simulink model "IncisionDicison"  (R2023a)
settings: Solver=FixedStepAuto  StartTime=0.0  StopTime=inf  RelTol=1e-3  EnableMultiTasking=on
libraries: vexarmcortexlib x24, vexcommonlib x7
settings Model: ExtModeTrigDuration=25  Creator=bobsi  LastModifiedBy=bobsi
settings OptimizationCC: EnhancedBackFolding=on  PassReuseOutputArgsAs=Individual arguments  ZeroExternalMemoryAtStartup=off  ZeroInternalMemoryAtStartup=off  MaxStackSize=64  OptimizeBlockOrder=speed  DifferentSizesBufferReuse=on  OptimizationCustomize=off  EfficientTunableParamExpr=on
settings DebuggingCC: ParameterTunabilityLossMsg=error
settings HardwareCC: ProdBitPerPointer=32  ProdBitPerSizeT=32  ProdBitPerPtrDiffT=32  ProdLargestAtomicInteger=Long  ProdLargestAtomicFloat=Double  ProdWordSize=32  ProdHWDeviceType=ARM Compatible->ARM Cortex
settings SFSimCC: MATLABDynamicMemAlloc=off
settings RTWCC: Description=Embedded Coder  SystemTargetFile=ert.tlc  HardwareBoard=ARM Cortex-based VEX Microcontroller  TLCOptions="-aInlineSetEventsForThisBaseRateFcn=TLC_FALSE -aSuppressMultiTaskScheduler=TLC_FALSE  -aRateBasedStepFcn=0"  TemplateMakefile=ert_default_tmf  Toolchain=GNU Tools for VEX ARM Cortex
settings CodeAppCC: ForceParamTrailComments=on  IgnoreCustomStorageClasses=off  OperatorAnnotations=on  SimulinkDataObjDesc=on  SFDataObjDesc=on  InsertBlockDesc=on
settings ERTTargetCC: ExtModeTransport=1  ExtModeMexFile=ext_serial_win32_comm

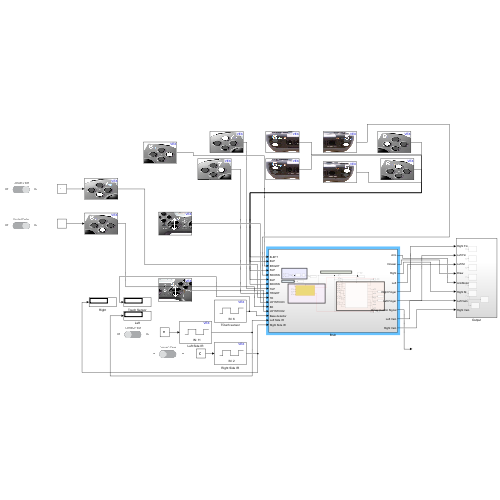
[thumbnail: Simulink's stored preview of the top-level diagram]
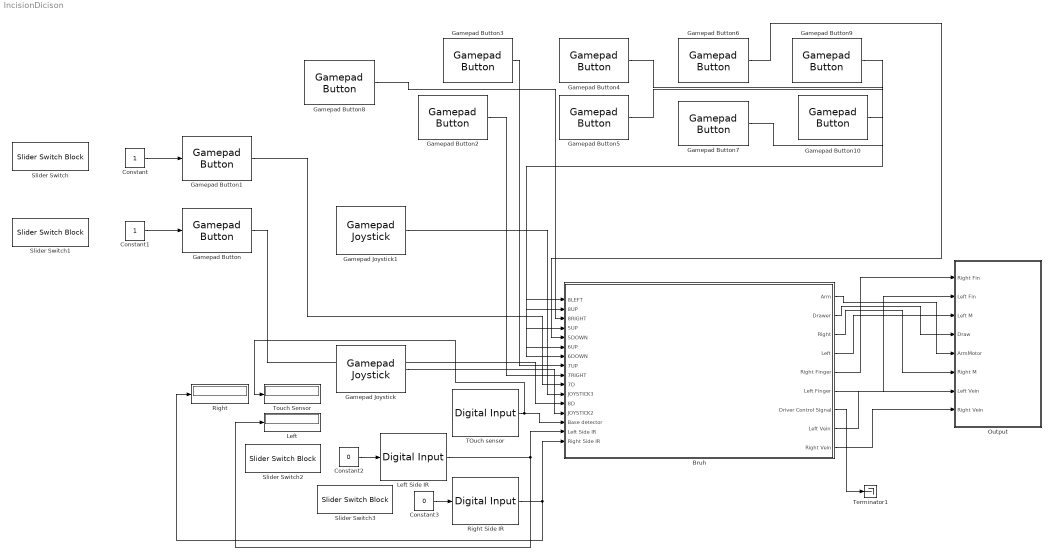
== system IncisionDicison ==
  Bruh : Subsystem
  Constant : Constant
  Constant1 : Constant
  Constant2 : Constant  Value=0
  Constant3 : Constant  Value=0
  Gamepad Button : vexarmcortexlib/Gamepad/Gamepad Button  joystick=1  chan=8  button56=Up  button78=Down  SimulationIn=on  SampleTime=0.02
  Gamepad Button1 : vexarmcortexlib/Gamepad/Gamepad Button  joystick=1  chan=7  button56=Up  button78=Down  SimulationIn=on  SampleTime=0.02
  Gamepad Button10 : vexarmcortexlib/Gamepad/Gamepad Button  joystick=1  chan=8  button56=Up  button78=Up  SimulationIn=off  SampleTime=0.02
  Gamepad Button2 : vexarmcortexlib/Gamepad/Gamepad Button  joystick=1  chan=7  button56=Up  button78=Right  SimulationIn=off  SampleTime=0.02
  Gamepad Button3 : vexarmcortexlib/Gamepad/Gamepad Button  joystick=1  chan=7  button56=Up  button78=Up  SimulationIn=off  SampleTime=0.02
  Gamepad Button4 : vexarmcortexlib/Gamepad/Gamepad Button  joystick=1  chan=6  button56=Down  button78=Down  SimulationIn=off  SampleTime=0.02
  Gamepad Button5 : vexarmcortexlib/Gamepad/Gamepad Button  joystick=1  chan=6  button56=Up  button78=Down  SimulationIn=off  SampleTime=0.02
  Gamepad Button6 : vexarmcortexlib/Gamepad/Gamepad Button  joystick=1  chan=5  button56=Down  button78=Down  SimulationIn=off  SampleTime=0.02
  Gamepad Button7 : vexarmcortexlib/Gamepad/Gamepad Button  joystick=1  chan=5  button56=Up  button78=Down  SimulationIn=off  SampleTime=0.02
  Gamepad Button8 : vexarmcortexlib/Gamepad/Gamepad Button  joystick=1  chan=8  button56=Up  button78=Right  SimulationIn=off  SampleTime=0.02
  Gamepad Button9 : vexarmcortexlib/Gamepad/Gamepad Button  joystick=1  chan=8  button56=Up  button78=Left  SimulationIn=off  SampleTime=0.02
  Gamepad Joystick : vexarmcortexlib/Gamepad/Gamepad Joystick  joystick=1  chan=2  SimulationIn=off  SampleTime=0.02
  Gamepad Joystick1 : vexarmcortexlib/Gamepad/Gamepad Joystick  joystick=1  chan=3  SimulationIn=off  SampleTime=0.02
  Left : Display
  Left Side IR : vexarmcortexlib/Sensors/Digital Input  inChan=11  SimulationIn=on  SampleTime=0.02
  Output : Subsystem
  Right : Display
  Right Side IR : vexarmcortexlib/Sensors/Digital Input  inChan=2  SimulationIn=on  SampleTime=0.02
  Slider Switch{,1..3} (4 alike) : SliderSwitchBlock
      settings: Values={{'Off', 'On'}, [0 1]}
  TOuch sensor : vexarmcortexlib/Sensors/Digital Input  inChan=6  SimulationIn=off  SampleTime=0.02
  Terminator1 : Terminator
  Touch Sensor : Display
  wires:
  Bruh/3(Right) -> Output/6(Right M)
  Bruh/6(Left Finger) -> Output/2(Left Fin)
  Bruh/5(Right Finger) -> Output/1(Right Fin)
  Bruh/4(Left) -> Output/3(Left M)
  Bruh/2(Drawer) -> Output/4(Draw)
  Bruh/1(Arm) -> Output/5(ArmMotor)
  Bruh/7(Driver Control Signal) -> Terminator1/1
  Right Side IR/1 -> Right/1, Bruh/16(Right Side IR)
  Left Side IR/1 -> Left/1, Bruh/15(Left Side IR)
  TOuch sensor/1 -> Touch Sensor/1, Bruh/14(Base detector)
  Gamepad Joystick/1 -> Bruh/13(JOYSTICK2)
  Gamepad Button/1 -> Bruh/12(8D)
  Gamepad Joystick1/1 -> Bruh/11(JOYSTICK3)
  Gamepad Button1/1 -> Bruh/10(7D)
  Gamepad Button2/1 -> Bruh/9(7RIGHT)
  Gamepad Button3/1 -> Bruh/8(7UP)
  Gamepad Button4/1 -> Bruh/7(6DOWN)
  Gamepad Button5/1 -> Bruh/6(6UP)
  Gamepad Button6/1 -> Bruh/5(5DOWN)
  Gamepad Button7/1 -> Bruh/4(5UP)
  Gamepad Button8/1 -> Bruh/3(8RIGHT)
  Gamepad Button10/1 -> Bruh/2(8UP)
  Gamepad Button9/1 -> Bruh/1(8LEFT)
  Bruh/8(Left Vein) -> Output/7(Left Vein)
  Bruh/9(Right Vein) -> Output/8(Right Vein)
  Constant/1 -> Gamepad Button1/1
  Constant1/1 -> Gamepad Button/1
  Constant2/1 -> Left Side IR/1
  Constant3/1 -> Right Side IR/1

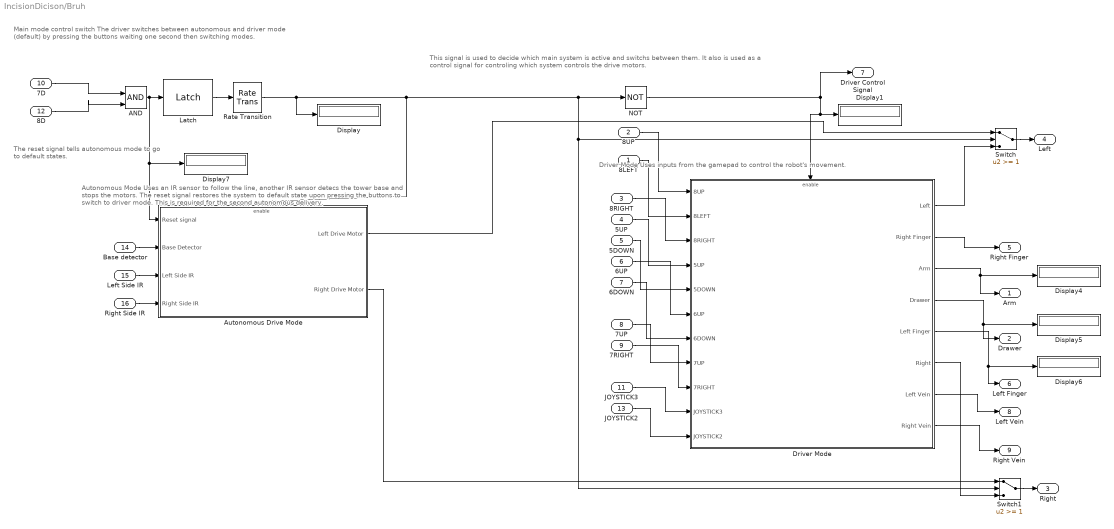
== system IncisionDicison/Bruh ==
  note: Driver Mode
      | Uses inputs from the gamepad to control the robot's movement.
  note: This signal is used to decide which main system is active and switchs between them.
      | It also is used as a control signal for controling which system controls the drive motors.
  note: The reset signal tells autonomous
      | mode to go to default states.
  note: Autonomous Mode
      | 	Uses an IR sensor to follow the line, another IR sensor detecs the
      | 	tower base and stops the motors. The reset signal restores the system
      | 	to default state upon pressing the buttons to switch to driver mode. This
      | 	is required for the second autonomous delivery.
  note: Main mode control switch
      | The driver switches between autonomous and driver mode (default) by
      | pressing the buttons waiting one second then switching modes.
  8LEFT : Inport
  8UP : Inport  Port=2
  8RIGHT : Inport  Port=3
  5UP : Inport  Port=4
  5DOWN : Inport  Port=5
  6UP : Inport  Port=6
  6DOWN : Inport  Port=7
  7UP : Inport  Port=8
  7RIGHT : Inport  Port=9
  7D : Inport  Port=10
  JOYSTICK3 : Inport  Port=11
  8D : Inport  Port=12
  JOYSTICK2 : Inport  Port=13
  Base detector : Inport  Port=14
  Left Side IR : Inport  Port=15
  Right Side IR : Inport  Port=16
  "AND " : Logic  IconShape=distinctive  AllPortsSameDT=off  OutDataTypeStr=boolean
  Autonomous Drive Mode : Subsystem
  Display{,1,4..7} (6 alike) : Display
  Driver Mode : Subsystem  TreatAsAtomicUnit=on
  Latch : vexcommonlib/Latch  output0=off  BlockPlatform=vexarmcortex
  NOT : Logic  Operator=NOT  IconShape=distinctive  AllPortsSameDT=off  OutDataTypeStr=boolean
  Rate Transition : RateTransition
  Switch : Switch  Threshold=1  SaturateOnIntegerOverflow=off  InputSameDT=off
  Switch1 : Switch  Threshold=1  SaturateOnIntegerOverflow=off  InputSameDT=off
  Arm : Outport
  Drawer : Outport  Port=2
  Right : Outport  Port=3
  Left : Outport  Port=4
  Right Finger : Outport  Port=5
  Left Finger : Outport  Port=6
  Driver Control Signal : Outport  Port=7
  Left Vein : Outport  Port=8
  Right Vein : Outport  Port=9
  wires:
  7D/1 -> "AND "/1
  "AND "/1 -> Latch/1, Display7/1, Autonomous Drive Mode/1(Reset signal)
  8D/1 -> "AND "/2
  Rate Transition/1 -> Display/1, Autonomous Drive Mode/Enable, NOT/1, Switch1/2, Switch/2
  NOT/1 -> Display1/1, Driver Mode/Enable, Driver Control Signal/1
  Autonomous Drive Mode/1(Left Drive Motor) -> Switch/1
  Switch/1 -> Left/1
  Autonomous Drive Mode/2(Right Drive Motor) -> Switch1/1
  Switch1/1 -> Right/1
  Left Side IR/1 -> Autonomous Drive Mode/3(Left Side IR)
  Base detector/1 -> Autonomous Drive Mode/2(Base Detector)
  7RIGHT/1 -> Driver Mode/9(7RIGHT)
  JOYSTICK3/1 -> Driver Mode/10(JOYSTICK3)
  JOYSTICK2/1 -> Driver Mode/11(JOYSTICK2)
  7UP/1 -> Driver Mode/8(7UP)
  Driver Mode/4(Drawer) -> Drawer/1, Display5/1
  Driver Mode/3(Arm) -> Arm/1, Display4/1
  Driver Mode/1(Left) -> Switch/3
  5DOWN/1 -> Driver Mode/5(5DOWN)
  5UP/1 -> Driver Mode/4(5UP)
  6UP/1 -> Driver Mode/6(6UP)
  6DOWN/1 -> Driver Mode/7(6DOWN)
  Right Side IR/1 -> Autonomous Drive Mode/4(Right Side IR)
  Latch/1 -> Rate Transition/1
  Driver Mode/6(Right) -> Switch1/3
  Driver Mode/5(Left Finger) -> Left Finger/1, Display6/1
  Driver Mode/2(Right Finger) -> Right Finger/1
  8RIGHT/1 -> Driver Mode/3(8RIGHT)
  8LEFT/1 -> Driver Mode/2(8LEFT)
  8UP/1 -> Driver Mode/1(8UP)
  Driver Mode/7(Left Vein) -> Left Vein/1
  Driver Mode/8(Right Vein) -> Right Vein/1

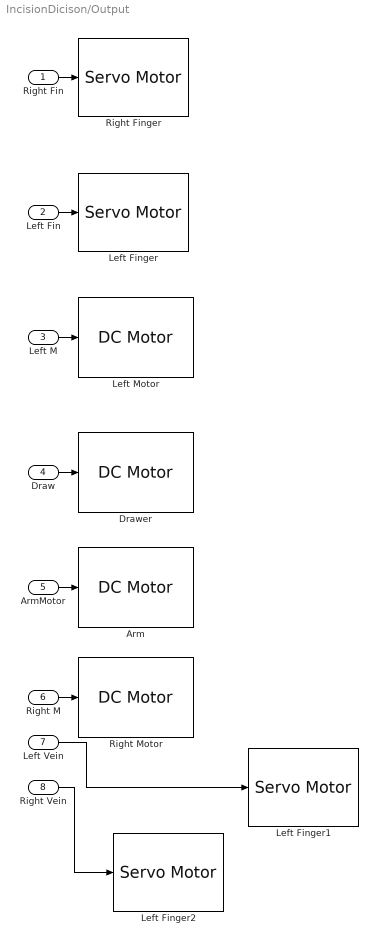
== system IncisionDicison/Output ==
  Right Fin : Inport
  Left Fin : Inport  Port=2
  Left M : Inport  Port=3
  Draw : Inport  Port=4
  ArmMotor : Inport  Port=5
  Right M : Inport  Port=6
  Left Vein : Inport  Port=7
  Right Vein : Inport  Port=8
  Arm : vexarmcortexlib/Actuators/DC Motor  motor=6  scaleFactor=1/13.5  SimulationOut=off
  Drawer : vexarmcortexlib/Actuators/DC Motor  motor=4  scaleFactor=1/13.5  SimulationOut=off
  Left Finger : vexarmcortexlib/Actuators/Servo Motor  motor=3  scaleFactor=60/127  SimulationOut=off
  Left Finger1 : vexarmcortexlib/Actuators/Servo Motor  motor=7  scaleFactor=60/127  SimulationOut=off
  Left Finger2 : vexarmcortexlib/Actuators/Servo Motor  motor=8  scaleFactor=60/127  SimulationOut=off
  Left Motor : vexarmcortexlib/Actuators/DC Motor  motor=2  scaleFactor=1/13.5  SimulationOut=off
  Right Finger : vexarmcortexlib/Actuators/Servo Motor  motor=5  scaleFactor=60/127  SimulationOut=off
  Right Motor : vexarmcortexlib/Actuators/DC Motor  motor=9  scaleFactor=1/13.5  SimulationOut=off
  wires:
  Right M/1 -> Right Motor/1
  Right Fin/1 -> Right Finger/1
  Draw/1 -> Drawer/1
  Left Fin/1 -> Left Finger/1
  ArmMotor/1 -> Arm/1
  Left M/1 -> Left Motor/1
  Left Vein/1 -> Left Finger1/1
  Right Vein/1 -> Left Finger2/1

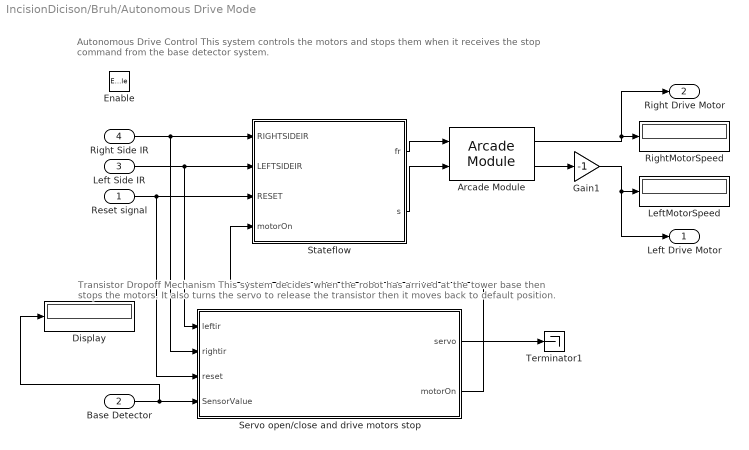
== system IncisionDicison/Bruh/Autonomous Drive Mode ==
  note: Transistor Dropoff Mechanism
      | This system decides when the robot has arrived at the tower base then stops the motors. It also turns the servo to
      | release the transistor then it moves back to default position.
  note: Autonomous Drive Control
      | This system controls the motors and stops them when it receives the stop command from the base detector system.
  Reset signal : Inport
  Base Detector : Inport  Port=2
  Left Side IR : Inport  Port=3
  Right Side IR : Inport  Port=4
  Enable : EnablePort
  Arcade Module : vexcommonlib/Arcade Module  BlockPlatform=vexarmcortex
  Display : Display
  Gain1 : Gain  Gain=-1
  LeftMotorSpeed : Display
  RightMotorSpeed : Display
  Servo open/close and drive motors stop : Stateflow chart  TreatAsAtomicUnit=on
  Stateflow : Stateflow chart  TreatAsAtomicUnit=on
  Terminator1 : Terminator
  Left Drive Motor : Outport
  Right Drive Motor : Outport  Port=2
  wires:
  Left Side IR/1 -> Servo open/close and drive motors stop/1(leftir), Stateflow/2(LEFTSIDEIR)
  Stateflow/2(s) -> Arcade Module/2
  Stateflow/1(fr) -> Arcade Module/1
  Reset signal/1 -> Stateflow/3(RESET), Servo open/close and drive motors stop/3(reset)
  Right Side IR/1 -> Servo open/close and drive motors stop/2(rightir), Stateflow/1(RIGHTSIDEIR)
  Servo open/close and drive motors stop/2(motorOn) -> Stateflow/4(motorOn)
  Servo open/close and drive motors stop/1(servo) -> Terminator1/1
  Arcade Module/2 -> Gain1/1
  Arcade Module/1 -> RightMotorSpeed/1, Right Drive Motor/1
  Base Detector/1 -> Display/1, Servo open/close and drive motors stop/4(SensorValue)
  Gain1/1 -> LeftMotorSpeed/1, Left Drive Motor/1

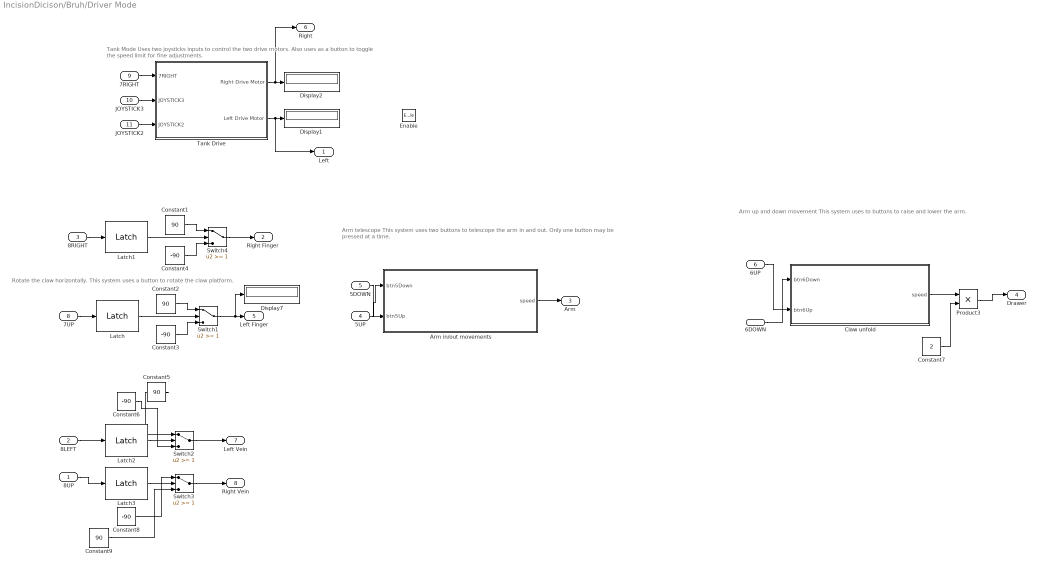
== system IncisionDicison/Bruh/Driver Mode ==
  note: Rotate the claw horizontally.
      | This system uses a button to rotate the claw platform.
  note: Tank Mode
      | Uses two joysticks inputs to control the two drive motors. Also uses as a button
      | to toggle the speed limit for fine adjustments.
  note: Arm telescope
      | This system uses two buttons to telescope the arm in and out.
      | Only one button may be pressed at a time.
  note: Arm up and down movement
      | This system uses to buttons to raise and lower the arm.
  8UP : Inport
  8LEFT : Inport  Port=2
  8RIGHT : Inport  Port=3
  5UP : Inport  Port=4
  5DOWN : Inport  Port=5
  6UP : Inport  Port=6
  6DOWN : Inport  Port=7
  7UP : Inport  Port=8
  7RIGHT : Inport  Port=9
  JOYSTICK3 : Inport  Port=10
  JOYSTICK2 : Inport  Port=11
  Enable : EnablePort
  Arm in/out movements : Stateflow chart  TreatAsAtomicUnit=on
  Claw unfold : Stateflow chart  TreatAsAtomicUnit=on
  Constant{1..2,5,9} (4 alike) : Constant  Value=90
  Constant{3..4,6,8} (4 alike) : Constant  Value=-90
  Constant7 : Constant  Value=2
  Display1 : Display
  Display2 : Display
  Display7 : Display
  Latch{,1..3} (4 alike) : vexcommonlib/Latch  output0=off  BlockPlatform=vexarmcortex
  Product3 : Product  RndMeth=Zero
  Switch{1..4} (4 alike) : Switch  Threshold=1  SaturateOnIntegerOverflow=off  InputSameDT=off
  "Tank Drive " : Subsystem  TreatAsAtomicUnit=on
  Left : Outport
  Right Finger : Outport  Port=2
  Arm : Outport  Port=3
  Drawer : Outport  Port=4
  Left Finger : Outport  Port=5
  Right : Outport  Port=6
  Left Vein : Outport  Port=7
  Right Vein : Outport  Port=8
  wires:
  JOYSTICK3/1 -> "Tank Drive "/2(JOYSTICK3)
  JOYSTICK2/1 -> "Tank Drive "/3(JOYSTICK2)
  7UP/1 -> Latch/1
  Latch/1 -> Switch1/2
  Switch1/1 -> Display7/1, Left Finger/1
  Constant2/1 -> Switch1/1
  Constant3/1 -> Switch1/3
  7RIGHT/1 -> "Tank Drive "/1(7RIGHT)
  "Tank Drive "/2(Left Drive Motor) -> Left/1, Display1/1
  "Tank Drive "/1(Right Drive Motor) -> Right/1, Display2/1
  6DOWN/1 -> Claw unfold/1(btn6Down)
  6UP/1 -> Claw unfold/2(btn6Up)
  Constant4/1 -> Switch4/3
  8RIGHT/1 -> Latch1/1
  Constant1/1 -> Switch4/1
  Latch1/1 -> Switch4/2
  Switch4/1 -> Right Finger/1
  Arm in/out movements/1(speed) -> Arm/1
  Claw unfold/1(speed) -> Product3/1
  Product3/1 -> Drawer/1
  Constant7/1 -> Product3/2
  5DOWN/1 -> Arm in/out movements/2(btn5Up)
  5UP/1 -> Arm in/out movements/1(btn5Down)
  8UP/1 -> Latch3/1
  8LEFT/1 -> Latch2/1
  Latch3/1 -> Switch3/2
  Latch2/1 -> Switch2/2
  Switch2/1 -> Left Vein/1
  Switch3/1 -> Right Vein/1
  Constant5/1 -> Switch2/1
  Constant6/1 -> Switch2/3
  Constant8/1 -> Switch3/1
  Constant9/1 -> Switch3/3

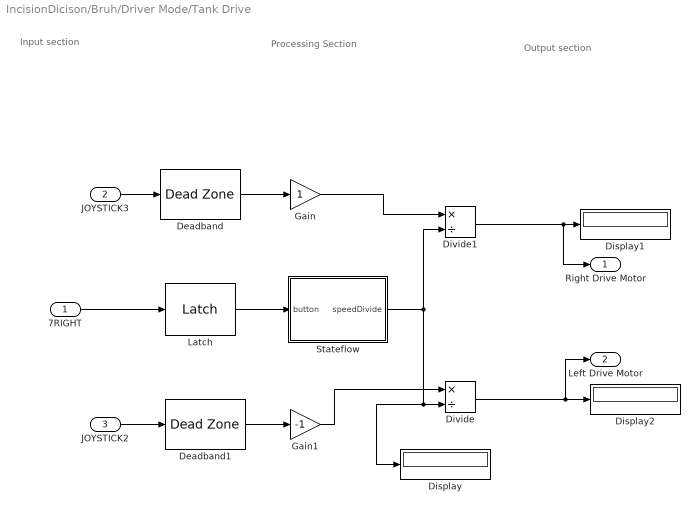
== system IncisionDicison/Bruh/Driver Mode/Tank Drive  ==
  note: Output section
  note: Processing Section
  note: Input section
  7RIGHT : Inport
  JOYSTICK3 : Inport  Port=2
  JOYSTICK2 : Inport  Port=3
  Deadband : DeadZone  LowerValue=-5  UpperValue=5
  Deadband1 : DeadZone  LowerValue=-5  UpperValue=5
  Display : Display
  Display1 : Display
  Display2 : Display
  Divide : Product  Inputs=*/
  Divide1 : Product  Inputs=*/
  Gain : Gain
  Gain1 : Gain  Gain=-1
  Latch : vexcommonlib/Latch  output0=off  BlockPlatform=vexarmcortex
  Stateflow : Stateflow chart  TreatAsAtomicUnit=on
  Right Drive Motor : Outport
  Left Drive Motor : Outport  Port=2
  wires:
  JOYSTICK3/1 -> Deadband/1
  7RIGHT/1 -> Latch/1
  Latch/1 -> Stateflow/1(button)
  Stateflow/1(speedDivide) -> Divide1/2, Display/1, Divide/2
  Deadband/1 -> Gain/1
  Divide1/1 -> Display1/1, Right Drive Motor/1
  JOYSTICK2/1 -> Deadband1/1
  Divide/1 -> Display2/1, Left Drive Motor/1
  Deadband1/1 -> Gain1/1
  Gain/1 -> Divide1/1
  Gain1/1 -> Divide/1

== stateflow chart IncisionDicison/Bruh/Driver Mode/Arm in//out movements ==
  state ARMDOWN
    entry:
    speed = -100;
  state STOPPED
    entry:
    speed = 30;
  state ARMUP
    entry:
    speed = 80;
  (default) -> STOPPED
  STOPPED -> ARMUP [order 1] : [btn5Down == 0 && btn5Up == 1 ]
  STOPPED -> ARMDOWN [order 2] : [btn5Down == 1 && btn5Up == 0]
  ARMDOWN -> STOPPED [order 2] : [btn5Down == 0]
  ARMUP -> STOPPED [order 2] : [btn5Up == 0]
  ARMDOWN -> STOPPED [order 1] : [btn5Down == 1 && btn5Up == 1]
  ARMUP -> STOPPED [order 1] : [btn5Down == 1 && btn5Up == 1]
  data: btn5Down input; btn5Up input; speed output

== stateflow chart IncisionDicison/Bruh/Driver Mode/Claw unfold ==
  state ARMDOWN
    entry:
    speed = -50;
  state STOPPED
    entry:
    speed = 0;
  state ARMUP
    entry:
    speed = 140;
  (default) -> STOPPED
  STOPPED -> ARMUP [order 1] : [btn6Down == 0 && btn6Up == 1 ]
  STOPPED -> ARMDOWN [order 2] : [btn6Down == 1 && btn6Up == 0]
  ARMDOWN -> STOPPED [order 2] : [btn6Down == 0]
  ARMUP -> STOPPED [order 2] : [btn6Up == 0]
  ARMDOWN -> STOPPED [order 1] : [btn6Down == 1 && btn6Up == 1]
  ARMUP -> STOPPED [order 1] : [btn6Down == 1 && btn6Up == 1]
  data: speed output; btn6Down input; btn6Up input

== stateflow chart IncisionDicison/Bruh/Autonomous Drive Mode/Stateflow ==
  state STRAIGHT
    entry:
    fr = 110;
    s = 0;
  state GO_RIGHT
    entry:
    fr = 90;
    s = 110;
  state GO_LEFT
    entry:
    fr = 90;
    s = -110;
  state BackUp
    entry:
    fr = -30;
    s = 30;
  state STOP
    entry:
    fr = 0;
    s = 0;
  (default) -> STRAIGHT
  GO_LEFT -> STRAIGHT [order 3] : [LEFTSIDEIR == 0 && RIGHTSIDEIR == 0]
  GO_RIGHT -> STRAIGHT [order 3] : [RIGHTSIDEIR == 0 && LEFTSIDEIR == 0]
  STRAIGHT -> GO_RIGHT [order 3] : [RIGHTSIDEIR == 0 && LEFTSIDEIR == 1]
  STRAIGHT -> GO_LEFT [order 2] : [LEFTSIDEIR == 0 && RIGHTSIDEIR ==1]
  STOP -> STRAIGHT [order 3] : [RIGHTSIDEIR == 0 && LEFTSIDEIR == 0 && RESET == 0]
  STRAIGHT -> STOP [order 1] : [motorOn == 0]
  GO_LEFT -> GO_RIGHT [order 2] : [LEFTSIDEIR == 1 && RIGHTSIDEIR == 0]
  GO_RIGHT -> GO_LEFT [order 2] : [RIGHTSIDEIR == 1 && LEFTSIDEIR == 0]
  STOP -> GO_LEFT [order 2] : [RESET == 0 && LEFTSIDEIR == 0]
  GO_LEFT -> STOP [order 1] : [motorOn == 0]
  STOP -> GO_RIGHT [order 1] : [RESET == 0 && RIGHTSIDEIR == 0]
  GO_RIGHT -> STOP [order 1] : [motorOn == 0]
  BackUp -> STOP : [motorOn == 2]
  STOP -> BackUp [order 4] : [motorOn ==2]
  data: RIGHTSIDEIR input; LEFTSIDEIR input; RESET input; motorOn input; fr output; s output

== stateflow chart IncisionDicison/Bruh/Driver Mode/Tank Drive /Stateflow ==
  state Full_Speed
    entry:
    speedDivide = 1
  state Slow_Speed
    entry:
    speedDivide = 2
  (default) -> Full_Speed
  Full_Speed -> Slow_Speed : [button]
  Slow_Speed -> Full_Speed : [button == 0]
  data: speedDivide output; button input

== stateflow chart IncisionDicison/Bruh/Autonomous Drive Mode/Servo open//close and drive motors stop ==
  state move
    entry:
    servo = 0;
    motorOn = 1;
  state off
    entry:
    servo = 0;
    motorOn = 0;
  (default) -> move
  move -> off : [SensorValue == 1]
  off -> move : [reset == 0 && SensorValue == 1 && leftir == 1 && rightir == 1]
  data: leftir input; rightir input; reset input; SensorValue input; servo output; motorOn output
